simulink model "controller_lonV"  (R2017b)
settings: Solver=VariableStepAuto  StartTime=0.0  StopTime=30  RelTol=1e-3
values from neighbouring files (symbols this model uses):
  CSim_Hdot = 0    [controller_lonV_design.m]    (also in lonV_gain20190526.mat)
  CSim_V = 1    [controller_lonV_design.m]
  KF_Hdot = 0    [controller_lonV_design.m]    (also in lonV_gain20190526.mat = 32.9391189734)
  KF_theta = 0    [controller_lonV_design.m]    (also in lonV_gain20190526.mat = 2.23542028928)
  KF_V = 0    [controller_lonV_design.m]    (also in lonV_gain20190526.mat = 1.22259697794)
  KI_Hdot = 0    [controller_lonV_design.m]    (also in lonV_gain20190526.mat = -11.0424311113)
  KI_theta = 0    [controller_lonV_design.m]    (also in lonV_gain20190526.mat = -2.68927731907e-08)
  KI_V = 0    [controller_lonV_design.m]    (also in lonV_gain20190526.mat = 0.051424669333)
  KP_Hdot = 1    [controller_lonV_design.m]    (also in lonV_gain20190526.mat = -40.2759129728)
  KP_q = 1    [controller_lonV_design.m]    (also in lonV_gain20190526.mat = 0.00125827206562)
  KP_q2 = 1    [controller_lonV_design.m]    (also in lonV_gain20190526.mat = 8.28535161215)
  KP_theta = 1    [controller_lonV_design.m]    (also in lonV_gain20190526.mat = -2.50433076124)
  KP_V = 1    [controller_lonV_design.m]    (also in lonV_gain20190526.mat = 18.7143390736)
  Tau_DE = 0.05    [controller_lonV_design.m]    (also in lonV_gain20190526.mat)
  Tau_DTHR = 0.1    [controller_lonV_design.m]
undefined symbols (not defined in the file or in its folder): Actuators, alphax, Linmod
settings Model: Creator=zht  LastModifiedBy=zht

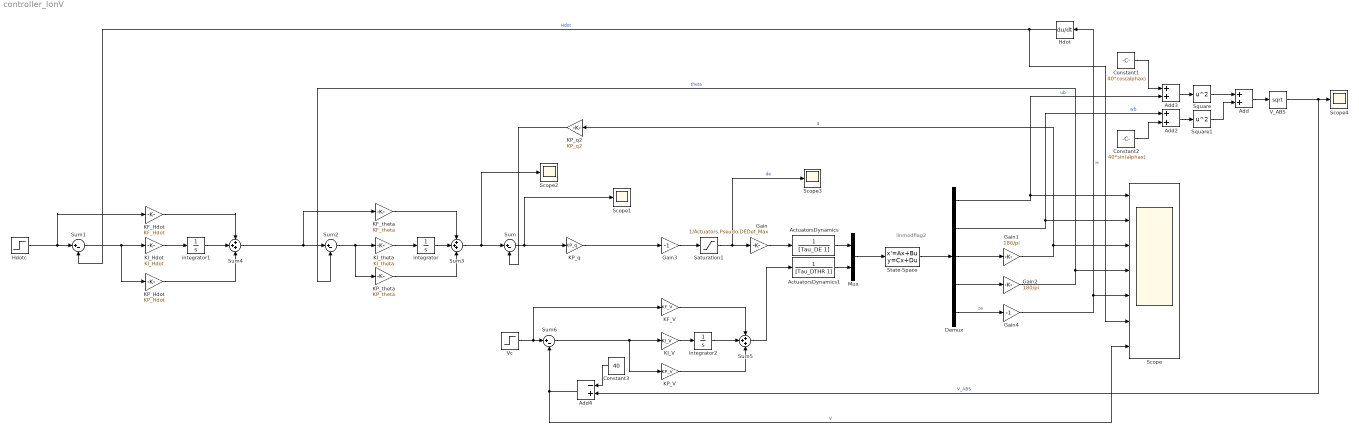
== system controller_lonV ==
  note: linmodflag2
  ActuatorsDynamics : TransferFcn  Denominator=[Tau_DE 1]
  ActuatorsDynamics1 : TransferFcn  Denominator=[Tau_DTHR 1]
  Add : Sum
  Add2 : Sum
  Add3 : Sum
  Add4 : Sum  Inputs=-+
  Constant1 : Constant  Value=40*cos(alphax)
  Constant2 : Constant  Value=40*sin(alphax)
  Constant3 : Constant  Value=40
  Demux : Demux  Outputs=5
  Gain : Gain  Gain=1/Actuators.Pseudo.DEDef_Max
  Gain1 : Gain  Gain=180/pi
  Gain2 : Gain  Gain=180/pi
  Gain3 : Gain  Gain=-1
  Gain4 : Gain  Gain=-1
  Hdot : Derivative  CoefficientInTFapproximation=0.0001
  Hdotc : Step  Time=0  After=CSim_Hdot  SampleTime=0
  KF_Hdot : Gain  Gain=KF_Hdot
  KF_V : Gain  Gain=KF_V
  KF_theta : Gain  Gain=KF_theta
  KI_Hdot : Gain  Gain=KI_Hdot
  KI_V : Gain  Gain=KI_V
  KI_theta : Gain  Gain=KI_theta
  KP_Hdot : Gain  Gain=KP_Hdot
  KP_V : Gain  Gain=KP_V
  KP_q : Gain  Gain=KP_q
  KP_q2 : Gain  Gain=KP_q2
  KP_theta : Gain  Gain=KP_theta
  Mux : Mux  Inputs=2
  Saturation1 : Saturate  UpperLimit=Actuators.Pseudo.DEDef_Max  LowerLimit=-Actuators.Pseudo.DEDef_Max
  Scope : Scope  NumInputPorts=7
  Scope{1..4} (4 alike) : Scope
  Square : Math  Operator=square  RndMeth=Zero  SaturateOnIntegerOverflow=on
  Square1 : Math  Operator=square  RndMeth=Zero  SaturateOnIntegerOverflow=on
  State-Space : StateSpace  A=Linmod.Lon_5.A  B=Linmod.Lon_5.B  C=Linmod.Lon_5.C  D=Linmod.Lon_5.D  InitialCondition=0  ContinuousStateAttributes={'ub','wb','q','theta','H'}
  Sum{,1..2,6} (4 alike) : Sum  Inputs=|+-
  Sum3 : Sum  Inputs=+++
  Sum4 : Sum  Inputs=+++
  Sum5 : Sum  Inputs=+++
  V_ABS : Sqrt  SaturateOnIntegerOverflow=on
  Vc : Step  Time=0  After=CSim_V  SampleTime=0
  integrator : Integrator
  integrator1 : Integrator
  integrator2 : Integrator
  wires:
  Mux/1 -> State-Space/1
  Sum6/1 -> KP_V/1, KI_V/1
  State-Space/1 -> Demux/1
  Demux/2 -> Add2/1, Scope/2  "wb"
  Demux/3 -> Gain1/1
  Demux/4 -> Gain2/1
  Demux/5 -> Gain4/1  "ze"
  Demux/1 -> Add3/2, Scope/1  "ub"
  Gain1/1 -> KP_q2/1, Scope/3  "q"
  Gain2/1 -> Sum2/2, Scope/4  "theta"
  Gain/1 -> ActuatorsDynamics/1
  Sum/1 -> KP_q/1, Scope1/1
  Sum3/1 -> Scope2/1, Sum/1
  Sum2/1 -> KP_theta/1, KI_theta/1
  KP_q2/1 -> Sum/2
  Saturation1/1 -> Scope3/1, Gain/1  "de"
  Gain3/1 -> Saturation1/1
  ActuatorsDynamics/1 -> Mux/1
  Sum1/1 -> KP_Hdot/1, KI_Hdot/1
  KP_q/1 -> Gain3/1
  integrator/1 -> Sum3/2
  KF_theta/1 -> Sum3/1
  KP_theta/1 -> Sum3/3
  KI_theta/1 -> integrator/1
  Hdot/1 -> Sum1/2, Scope/6  "Hdot"
  Sum4/1 -> KF_theta/1, Sum2/1
  KI_Hdot/1 -> integrator1/1
  Hdotc/1 -> KF_Hdot/1, Sum1/1
  KP_Hdot/1 -> Sum4/3
  integrator1/1 -> Sum4/2
  KF_Hdot/1 -> Sum4/1
  Gain4/1 -> Hdot/1, Scope/5  "H"
  Sum5/1 -> ActuatorsDynamics1/1
  KI_V/1 -> integrator2/1
  ActuatorsDynamics1/1 -> Mux/2
  Square/1 -> Add/1
  Square1/1 -> Add/2
  Add/1 -> V_ABS/1
  V_ABS/1 -> Add4/2, Scope4/1  "V_ABS"
  Vc/1 -> KF_V/1, Sum6/1
  Add2/1 -> Square1/1
  Constant2/1 -> Add2/2
  Add3/1 -> Square/1
  Constant1/1 -> Add3/1
  Constant3/1 -> Add4/1
  Add4/1 -> Scope/7, Sum6/2  "V"
  integrator2/1 -> Sum5/2
  KP_V/1 -> Sum5/3
  KF_V/1 -> Sum5/1
